simulink model "simFile"  (R2021a)
settings: Solver=VariableStepAuto  StartTime=0.0  StopTime=t(end)  MaxStep=TsH/10  RelTol=1e-3
values from neighbouring files (symbols this model uses):
  Pdt = ss(c2d(G,TsH,'tustin'))    [MultiRateLPM.m]    (also in MultiratePFG.m = ss(c2d(G,TsH)))
  TsH = 1/fs    (= 0.004)    [MRStandardPlantLPMExample.m]    (also in MultiRateLPM.m = 0.005; MultiratePFG.m = 0.005; unliftfrd.m = TsL/F; unliftfrdWithoutRep.m = GliftSIMO.Ts)
  TsL = 1/fsL    (= 0.04)    [MRStandardPlantLPMExample.m]    (also in MultiRateLPM.m = 0.01; MultiratePFG.m = 0.01; unliftfrd.m = GliftSIMO.Ts)
undefined symbols (not defined in the file or in its folder): PdtH
libraries: simulink x1, dspsrcs4 x1
settings Model: Creator=s152009  LastModifiedBy=s152009

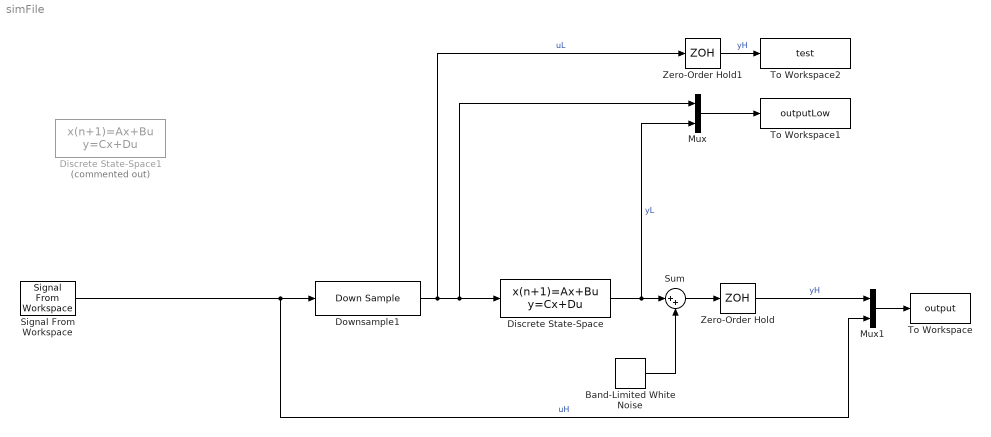
== system simFile ==
  Band-Limited White Noise : simulink/Sources/Band-Limited White Noise  Cov=[0.01]  Ts=TsL  seed=[23341]
  Discrete State-Space : DiscreteStateSpace  A=Pdt.A  B=Pdt.B  C=Pdt.C  D=Pdt.D  SampleTime=TsL
  Discrete State-Space1 : DiscreteStateSpace  Commented=on  A=PdtH.A  B=PdtH.B  C=PdtH.C  D=PdtH.D  SampleTime=TsH
  Downsample1 : DownSample  N=TsL/TsH  RateOptions=Allow multirate processing
  Mux : Mux  Inputs=2
  Mux1 : Mux  Inputs=2
  Signal From Workspace : dspsrcs4/Signal From Workspace  X=uH  Ts=TsH  nsamps=1  OutputAfterFinalValue=Setting to zero  ignoreOrWarnInputAndFrameLengths=off  OutputFrames=off
  Sum : Sum  Inputs=|++
  To Workspace : ToWorkspace  VariableName=output  SampleTime=-1
      settings: Save2DSignal=2-D array (concatenate along first dimension)
  To Workspace1 : ToWorkspace  VariableName=outputLow  SampleTime=-1
      settings: Save2DSignal=2-D array (concatenate along first dimension)
  To Workspace2 : ToWorkspace  VariableName=test  SampleTime=TsH
      settings: Save2DSignal=2-D array (concatenate along first dimension)
  Zero-Order Hold : ZeroOrderHold  SampleTime=TsH
  Zero-Order Hold1 : ZeroOrderHold  SampleTime=TsH
  wires:
  Discrete State-Space/1 -> Mux/2, Sum/1  "yL"
  Mux/1 -> To Workspace1/1
  Downsample1/1 -> Zero-Order Hold1/1, Mux/1, Discrete State-Space/1  "uL"
  Sum/1 -> Zero-Order Hold/1
  Band-Limited White Noise/1 -> Sum/2
  Signal From Workspace/1 -> Mux1/2, Downsample1/1  "uH"
  Mux1/1 -> To Workspace/1
  Zero-Order Hold/1 -> Mux1/1  "yH"
  Zero-Order Hold1/1 -> To Workspace2/1  "yH"
